simulink model "R2018a_AccBasedControl"  (R2018a)
settings: Solver=VariableStepAuto  StartTime=0.0  StopTime=10  RelTol=1e-3
libraries: simulink x2
settings Model: Creator=leonardof  LastModifiedBy=leonardof

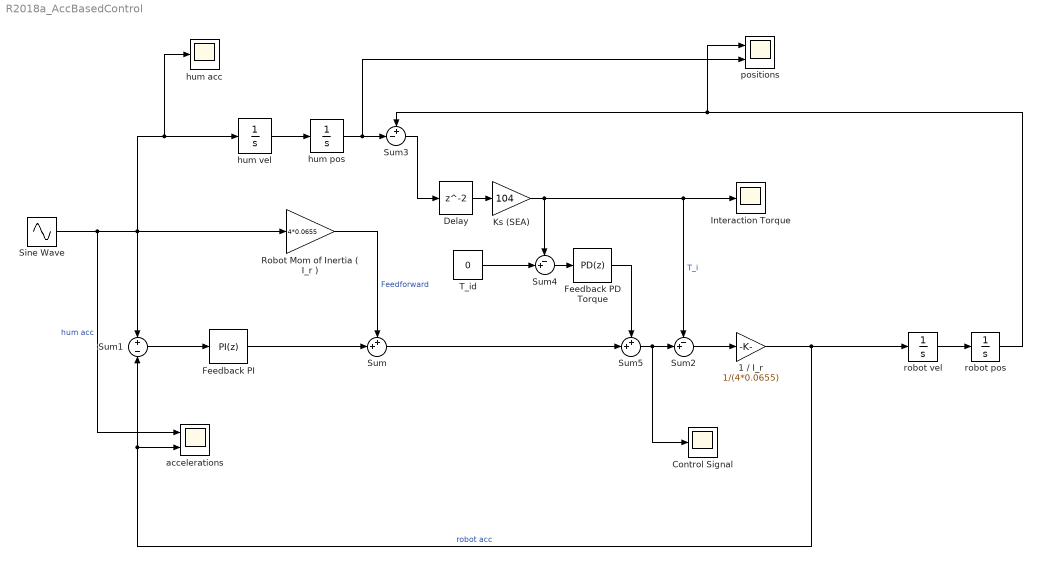
== system R2018a_AccBasedControl ==
  1 / I_r : Gain  Gain=1/(4*0.0655)
  Control Signal : Scope
  Delay : Delay  InitialCondition=0
  Feedback PD Torque : simulink/Continuous/PID Controller  Controller=PD  TimeDomain=Discrete-time  SampleTime=-1  IntegratorMethod=Forward Euler  FilterMethod=Forward Euler  Form=Parallel  UseFilter=on  ControllerParametersSource=internal  P=2.16249323632294  I=1  D=1.47040854354048  N=207.367614663794  InitialConditionSource=internal  InitialConditionForIntegrator=0  InitialConditionForFilter=0  ExternalReset=none  LimitOutput=off  UpperSaturationLimit=inf  LowerSaturationLimit=-inf  LinearizeAsGain=off  AntiWindupMode=none  Kb=1  TrackingMode=off  Kt=1  PParamMin=[]  PParamMax=[]  IParamMin=[]  IParamMax=[]  DParamMin=[]  DParamMax=[]  NParamMin=[]  NParamMax=[]  KbParamMin=[]  KbParamMax=[]  KtParamMin=[]  KtParamMax=[]  POutMin=[]  POutMax=[]  IOutMin=[]  IOutMax=[]  DOutMin=[]  DOutMax=[]  NOutMin=[]  NOutMax=[]  KbOutMin=[]  KbOutMax=[]  KtOutMin=[]  KtOutMax=[]  IntegratorOutMin=[]  IntegratorOutMax=[]  FilterOutMin=[]  FilterOutMax=[]  SumOutMin=[]  SumOutMax=[]  SumI1OutMin=[]  SumI1OutMax=[]  SumI2OutMin=[]  SumI2OutMax=[]  SumI3OutMin=[]  SumI3OutMax=[]  SumDOutMin=[]  SumDOutMax=[]  SaturationOutMin=[]  SaturationOutMax=[]  IntegratorContinuousStateAttributes=''  IntegratorStateMustResolveToSignalObject=off  IntegratorRTWStateStorageClass=Auto  FilterContinuousStateAttributes='torque'  FilterStateMustResolveToSignalObject=off  FilterRTWStateStorageClass=Auto  DifferentiatorICPrevScaledInput=0  DifferentiatorOutMin=[]  DifferentiatorOutMax=[]  FilterDiffOutCoefMin=[]  FilterDiffOutCoefMax=[]  SumDenOutMin=[]  SumDenOutMax=[]  SumNumOutMin=[]  SumNumOutMax=[]  ReciprocalOutMin=[]  ReciprocalOutMax=[]  DivideOutMin=[]  DivideOutMax=[]  TunerSelectOption=Transfer Function Based (PID Tuner App)
  Feedback PI : simulink/Continuous/PID Controller  Controller=PI  TimeDomain=Discrete-time  SampleTime=0.008333  IntegratorMethod=Forward Euler  FilterMethod=Forward Euler  Form=Parallel  UseFilter=on  ControllerParametersSource=internal  P=11.8522404144338  I=3.11402368205713  D=0  N=100  InitialConditionSource=internal  InitialConditionForIntegrator=0  InitialConditionForFilter=0  ExternalReset=none  LimitOutput=off  UpperSaturationLimit=inf  LowerSaturationLimit=-inf  LinearizeAsGain=off  AntiWindupMode=none  Kb=1  TrackingMode=off  Kt=1  PParamMin=[]  PParamMax=[]  IParamMin=[]  IParamMax=[]  DParamMin=[]  DParamMax=[]  NParamMin=[]  NParamMax=[]  KbParamMin=[]  KbParamMax=[]  KtParamMin=[]  KtParamMax=[]  POutMin=[]  POutMax=[]  IOutMin=[]  IOutMax=[]  DOutMin=[]  DOutMax=[]  NOutMin=[]  NOutMax=[]  KbOutMin=[]  KbOutMax=[]  KtOutMin=[]  KtOutMax=[]  IntegratorOutMin=[]  IntegratorOutMax=[]  FilterOutMin=[]  FilterOutMax=[]  SumOutMin=[]  SumOutMax=[]  SumI1OutMin=[]  SumI1OutMax=[]  SumI2OutMin=[]  SumI2OutMax=[]  SumI3OutMin=[]  SumI3OutMax=[]  SumDOutMin=[]  SumDOutMax=[]  SaturationOutMin=[]  SaturationOutMax=[]  IntegratorContinuousStateAttributes=''  IntegratorStateMustResolveToSignalObject=off  IntegratorRTWStateStorageClass=Auto  FilterContinuousStateAttributes=''  FilterStateMustResolveToSignalObject=off  FilterRTWStateStorageClass=Auto  DifferentiatorICPrevScaledInput=0  DifferentiatorOutMin=[]  DifferentiatorOutMax=[]  FilterDiffOutCoefMin=[]  FilterDiffOutCoefMax=[]  SumDenOutMin=[]  SumDenOutMax=[]  SumNumOutMin=[]  SumNumOutMax=[]  ReciprocalOutMin=[]  ReciprocalOutMax=[]  DivideOutMin=[]  DivideOutMax=[]  TunerSelectOption=Transfer Function Based (PID Tuner App)
  Interaction Torque : Scope
  Ks (SEA) : Gain  Gain=104
  "Robot Mom of Inertia ( I_r ) " : Gain  Gain=4*0.0655
  Sine Wave : Sin  Amplitude=40  Frequency=6.28318  SampleTime=0
  Sum : Sum  Inputs=++|
  Sum1 : Sum  Inputs=+|-
  Sum2 : Sum  Inputs=-+|
  Sum3 : Sum  Inputs=+-|
  Sum4 : Sum  Inputs=-+|
  Sum5 : Sum  Inputs=++|
  T_id : Constant  Value=0
  accelerations : Scope  NumInputPorts=2
  hum acc : Scope
  hum pos : Integrator  UpperSaturationLimit=1  LowerSaturationLimit=-1  ContinuousStateAttributes='position'
  hum vel : Integrator  InitialCondition=-40/6.28318  UpperSaturationLimit=20  LowerSaturationLimit=-20  ContinuousStateAttributes='velocity'
  positions : Scope  NumInputPorts=2
  robot pos : Integrator  UpperSaturationLimit=1  LowerSaturationLimit=-1  ContinuousStateAttributes='position'
  robot vel : Integrator  InitialCondition=-40/6.28318  UpperSaturationLimit=20  LowerSaturationLimit=-20  ContinuousStateAttributes='velocity'
  wires:
  Sine Wave/1 -> accelerations/1, hum acc/1, hum vel/1, Sum1/1, "Robot Mom of Inertia ( I_r ) "/1  "hum acc"
  "Robot Mom of Inertia ( I_r ) "/1 -> Sum/1  "Feedforward"
  Sum2/1 -> 1 / I_r/1
  1 / I_r/1 -> accelerations/2, Sum1/2, robot vel/1  "robot acc"
  hum vel/1 -> hum pos/1
  robot vel/1 -> robot pos/1
  hum pos/1 -> positions/2, Sum3/2
  Ks (SEA)/1 -> Sum4/1, Interaction Torque/1, Sum2/1  "T_i"
  robot pos/1 -> positions/1, Sum3/1
  Feedback PI/1 -> Sum/2
  Sum1/1 -> Feedback PI/1
  T_id/1 -> Sum4/2
  Sum4/1 -> Feedback PD Torque/1
  Feedback PD Torque/1 -> Sum5/1
  Sum5/1 -> Control Signal/1, Sum2/2
  Sum/1 -> Sum5/2
  Delay/1 -> Ks (SEA)/1
  Sum3/1 -> Delay/1
